simulink model "Main_EntryPoint"  (R2024b)
settings: Solver=VariableStepAuto  StartTime=0.0  StopTime=10.0  RelTol=1e-3
(part 1 of 2)
settings Model: Creator=The MathWorks, Inc.  LastModifiedBy=mitac
settings SolverCC: AlgebraicLoopSolver=TrustRegion
settings DataIOCC: ReturnWorkspaceOutputs=off
settings OptimizationCC: DefaultParameterBehavior=Inlined  ReuseModelBlockBuffer=off
settings DebuggingCC: UnconnectedInputMsg=warning  UnconnectedOutputMsg=warning  UnconnectedLineMsg=warning  ArithmeticOperatorsInVariantConditions=warning
settings ModelReferenceCC: EnableRefExpFcnMdlSchedulingChecks=on
settings SFSimCC: SimUseLocalCustomCode=off  CustomCodeUndefinedFunction=UseInterfaceOnly
settings RTWCC: RTWUseLocalCustomCode=off  GPUComputeCapability=3.5
settings CodeAppCC: StateflowObjectComments=on
settings ConfigComp: PLC_TargetIDE=HIMA_MITAC_1  PLC_MultiTBSigbuilderTimeRange=off  PLC_PreserveAliasType=on  PLC_GenerateReusableCode=on  PLC_FoldFBCallOutputVar=off  PLC_RemoveUnusedSSMethodCallArguments=on  PLC_FBUseSubsystemInstanceName=on  PLC_RemoveTopFBSSMethodType=on  PLC_UseCallOutputArgSyntax=on  PLC_OverrideDefaultNameLength=on  PLC_EnableUnsignedAndDoubleTypes=off  PLC_EnableUDTSplitting=off  PLC_MaxFieldsInUDT=500  PLC_InlineEnumCastFunction=off  PLC_RTWMaxIdLength=100  PLC_PreventExternalVarInitialization=on

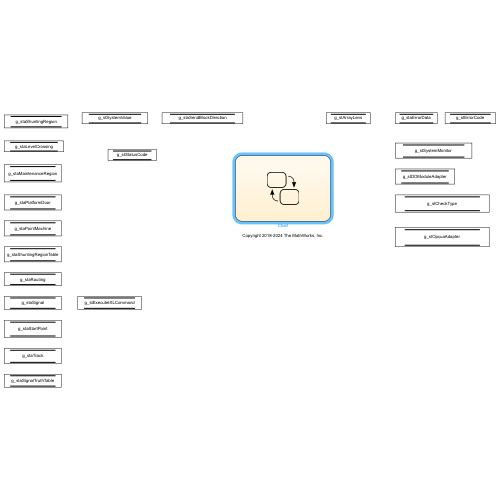
[thumbnail: Simulink's stored preview of the top-level diagram]
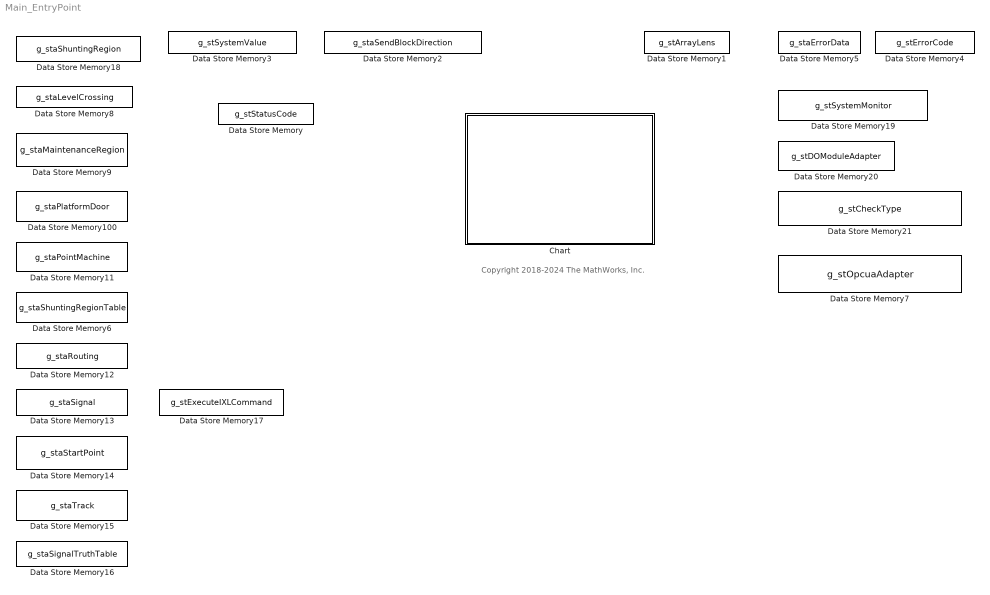
== system Main_EntryPoint ==
  note: Copyright 2018-2024 The MathWorks, Inc.
  Chart : Stateflow chart  TreatAsAtomicUnit=on
  Data Store Memory : DataStoreMemory  DataStoreName=g_stStatusCode  WriteAfterWriteMsg=warning  ShowAdditionalParam=off  OutDataTypeStr=Bus: ST_StatusCode  StateMustResolveToSignalObject=on
  Data Store Memory1 : DataStoreMemory  DataStoreName=g_stArrayLens  WriteAfterWriteMsg=warning  ShowAdditionalParam=off  OutDataTypeStr=Bus: ST_ArrayLens  StateMustResolveToSignalObject=on
  Data Store Memory100 : DataStoreMemory  DataStoreName=g_staPlatformDoor  WriteAfterWriteMsg=warning  ShowAdditionalParam=off  OutDataTypeStr=Bus: ST_PlatformDoor  Dimensions=16  StateMustResolveToSignalObject=on
  Data Store Memory11 : DataStoreMemory  DataStoreName=g_staPointMachine  WriteAfterWriteMsg=warning  ShowAdditionalParam=off  OutDataTypeStr=Bus: ST_PointMachine  Dimensions=36  StateMustResolveToSignalObject=on
  Data Store Memory12 : DataStoreMemory  DataStoreName=g_staRouting  WriteAfterWriteMsg=warning  ShowAdditionalParam=off  OutDataTypeStr=Bus: ST_Routing  Dimensions=96  StateMustResolveToSignalObject=on
  Data Store Memory13 : DataStoreMemory  DataStoreName=g_staSignal  WriteAfterWriteMsg=warning  ShowAdditionalParam=off  OutDataTypeStr=Bus: ST_Signal  Dimensions=36  StateMustResolveToSignalObject=on
  Data Store Memory14 : DataStoreMemory  DataStoreName=g_staStartPoint  WriteAfterWriteMsg=warning  ShowAdditionalParam=off  OutDataTypeStr=Bus: ST_StartPoint  Dimensions=16  StateMustResolveToSignalObject=on
  Data Store Memory15 : DataStoreMemory  DataStoreName=g_staTrack  WriteAfterWriteMsg=warning  ShowAdditionalParam=off  OutDataTypeStr=Bus: ST_Track  Dimensions=48  StateMustResolveToSignalObject=on
  Data Store Memory16 : DataStoreMemory  DataStoreName=g_staSignalTruthTable  WriteAfterWriteMsg=warning  ShowAdditionalParam=off  OutDataTypeStr=Bus: ST_SignalTruthTable  Dimensions=31  StateMustResolveToSignalObject=on
  Data Store Memory17 : DataStoreMemory  DataStoreName=g_stExecuteIXLCommand  WriteAfterWriteMsg=warning  ShowAdditionalParam=off  OutDataTypeStr=Bus: ST_IXLCommand  StateMustResolveToSignalObject=on
  Data Store Memory18 : DataStoreMemory  DataStoreName=g_staShuntingRegion  WriteAfterWriteMsg=warning  ShowAdditionalParam=off  OutDataTypeStr=Bus: ST_ShuntingRegion  Dimensions=16  StateMustResolveToSignalObject=on
  Data Store Memory19 : DataStoreMemory  DataStoreName=g_stSystemMonitor  WriteAfterWriteMsg=warning  ShowAdditionalParam=off  OutDataTypeStr=Bus: ST_SystemMonitor  StateMustResolveToSignalObject=on
  Data Store Memory2 : DataStoreMemory  DataStoreName=g_staSendBlockDirection  WriteAfterWriteMsg=warning  ShowAdditionalParam=off  OutDataTypeStr=Bus: ST_BlockDirection  Dimensions=8  StateMustResolveToSignalObject=on
  Data Store Memory20 : DataStoreMemory  DataStoreName=g_stDOModuleAdapter  WriteAfterWriteMsg=warning  ShowAdditionalParam=off  OutDataTypeStr=Bus: ST_DOModuleAdapter  Dimensions=1  StateMustResolveToSignalObject=on
  Data Store Memory21 : DataStoreMemory  DataStoreName=g_stCheckType  WriteAfterWriteMsg=warning  ShowAdditionalParam=off  OutDataTypeStr=Bus: ST_CheckType  StateMustResolveToSignalObject=on
  Data Store Memory3 : DataStoreMemory  DataStoreName=g_stSystemValue  WriteAfterWriteMsg=warning  ShowAdditionalParam=off  OutDataTypeStr=Bus: ST_SystemValue  StateMustResolveToSignalObject=on
  Data Store Memory4 : DataStoreMemory  DataStoreName=g_stErrorCode  WriteAfterWriteMsg=warning  ShowAdditionalParam=off  OutDataTypeStr=Bus: ST_ErrorCode  StateMustResolveToSignalObject=on
  Data Store Memory5 : DataStoreMemory  DataStoreName=g_staErrorData  WriteAfterWriteMsg=warning  ShowAdditionalParam=off  OutDataTypeStr=Bus: ST_ErrorData  Dimensions=100  StateMustResolveToSignalObject=on
  Data Store Memory6 : DataStoreMemory  DataStoreName=g_staShuntingRegionTable  WriteAfterWriteMsg=warning  ShowAdditionalParam=off  OutDataTypeStr=Bus: ST_ShuntingRegionTable  Dimensions=16  StateMustResolveToSignalObject=on
  Data Store Memory7 : DataStoreMemory  DataStoreName=g_stOpcuaAdapter  WriteAfterWriteMsg=warning  ShowAdditionalParam=off  OutDataTypeStr=Bus: ST_OPCUA_Adapter  StateMustResolveToSignalObject=on
  Data Store Memory8 : DataStoreMemory  DataStoreName=g_staLevelCrossing  WriteAfterWriteMsg=warning  ShowAdditionalParam=off  OutDataTypeStr=Bus: ST_LevelCrossing  Dimensions=8  StateMustResolveToSignalObject=on
  Data Store Memory9 : DataStoreMemory  DataStoreName=g_staMaintenanceRegion  WriteAfterWriteMsg=warning  ShowAdditionalParam=off  OutDataTypeStr=Bus: ST_MaintenanceRegion  Dimensions=16  StateMustResolveToSignalObject=on
